simulink model "actuator_models"  (R2024b)
settings: Solver=FixedStepAuto  StartTime=0.0  StopTime=3  FixedStep=0.0001  RelTol=1e-3
libraries: aerolibactuator x4
settings Model: Creator=jonno  LastModifiedBy=jonno

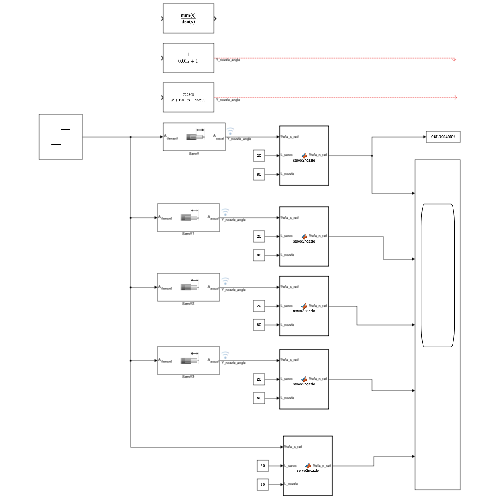
[thumbnail: Simulink's stored preview of the top-level diagram]
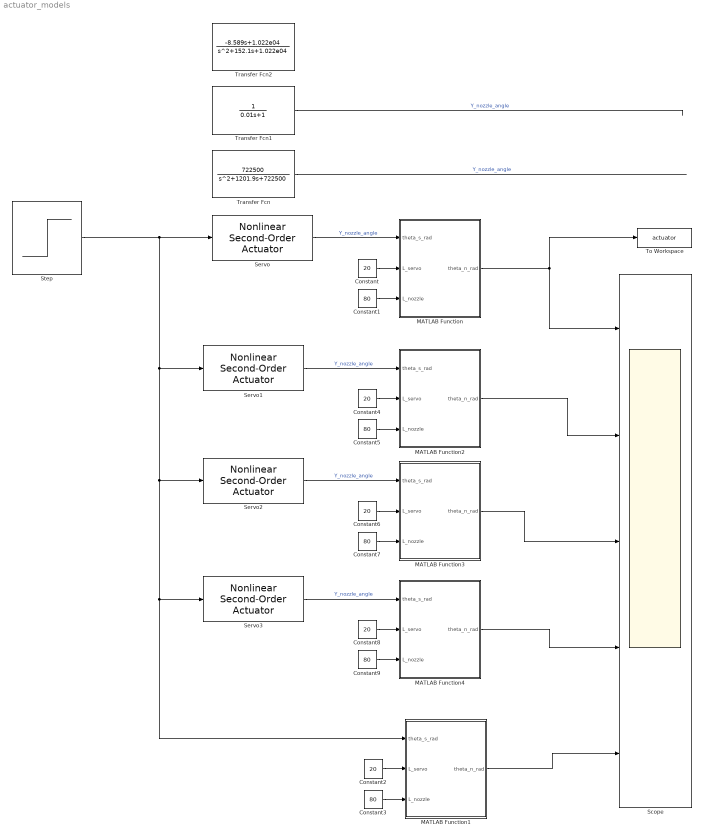
== system actuator_models ==
  Constant{,2,4,6,8} (5 alike) : Constant  Value=20
  Constant{1,3,5,7,9} (5 alike) : Constant  Value=80
  MATLAB Function : MATLAB Function  TreatAsAtomicUnit=on
  MATLAB Function1 : MATLAB Function  TreatAsAtomicUnit=on
  MATLAB Function2 : MATLAB Function  TreatAsAtomicUnit=on
  MATLAB Function3 : MATLAB Function  TreatAsAtomicUnit=on
  MATLAB Function4 : MATLAB Function  TreatAsAtomicUnit=on
  Scope : Scope  NumInputPorts=5
  Servo : aerolibactuator/Nonlinear Second-Order Actuator  wn_fin=60*10  z_fin=0.707  fin_max=60*pi/180  fin_min=-60*pi/180  fin_maxrate=(300*pi/180)*10  fin_act_0=0  fin_act_vel=0
  Servo1 : aerolibactuator/Nonlinear Second-Order Actuator  wn_fin=60*1  z_fin=0.707  fin_max=60*pi/180  fin_min=-60*pi/180  fin_maxrate=(300*pi/180)*10  fin_act_0=0  fin_act_vel=0
  Servo2 : aerolibactuator/Nonlinear Second-Order Actuator  wn_fin=60*10  z_fin=0.707  fin_max=60*pi/180  fin_min=-60*pi/180  fin_maxrate=(300*pi/180)*1  fin_act_0=0  fin_act_vel=0
  Servo3 : aerolibactuator/Nonlinear Second-Order Actuator  wn_fin=60*1  z_fin=0.707  fin_max=60*pi/180  fin_min=-60*pi/180  fin_maxrate=(300*pi/180)*1  fin_act_0=0  fin_act_vel=0
  Step : Step  Time=2  After=0.87266  SampleTime=0
  To Workspace : ToWorkspace  VariableName=actuator  SaveFormat=Timeseries  SampleTime=-1
  Transfer Fcn : TransferFcn  Numerator=[722500]  Denominator=[1 1201.9 722500]
  Transfer Fcn1 : TransferFcn  Denominator=[0.01 1]
  Transfer Fcn2 : TransferFcn  Numerator=[-8.589 1.022e04]  Denominator=[1 152.1 1.022e04]
  wires:
  Step/1 -> Servo1/1, Servo3/1, MATLAB Function1/1(theta_s_rad), Servo2/1, Servo/1
  Transfer Fcn/1 -> ?  "Y_nozzle_angle"
  Servo/1 -> MATLAB Function/1(theta_s_rad)  "Y_nozzle_angle"
  Transfer Fcn1/1 -> ?  "Y_nozzle_angle"
  MATLAB Function/1(theta_n_rad) -> To Workspace/1, Scope/1
  Constant/1 -> MATLAB Function/2(L_servo)
  Constant1/1 -> MATLAB Function/3(L_nozzle)
  Constant3/1 -> MATLAB Function1/3(L_nozzle)
  Constant2/1 -> MATLAB Function1/2(L_servo)
  MATLAB Function1/1(theta_n_rad) -> Scope/5
  Constant5/1 -> MATLAB Function2/3(L_nozzle)
  Servo1/1 -> MATLAB Function2/1(theta_s_rad)  "Y_nozzle_angle"
  MATLAB Function2/1(theta_n_rad) -> Scope/2
  Constant4/1 -> MATLAB Function2/2(L_servo)
  Constant6/1 -> MATLAB Function3/2(L_servo)
  Constant7/1 -> MATLAB Function3/3(L_nozzle)
  Servo2/1 -> MATLAB Function3/1(theta_s_rad)  "Y_nozzle_angle"
  Constant9/1 -> MATLAB Function4/3(L_nozzle)
  Constant8/1 -> MATLAB Function4/2(L_servo)
  Servo3/1 -> MATLAB Function4/1(theta_s_rad)  "Y_nozzle_angle"
  MATLAB Function3/1(theta_n_rad) -> Scope/3
  MATLAB Function4/1(theta_n_rad) -> Scope/4

== matlab function actuator_models/MATLAB Function ==
  data: theta_s_rad input; theta_n_rad output; L_servo input; L_nozzle input
function theta_n_rad = servo2nozzle(theta_s_rad, L_servo, L_nozzle)
    theta_n_rad = asin((L_servo / L_nozzle) * sin(theta_s_rad));
end

== matlab function actuator_models/MATLAB Function2 ==
  data: theta_s_rad input; theta_n_rad output; L_servo input; L_nozzle input
function theta_n_rad = servo2nozzle(theta_s_rad, L_servo, L_nozzle)
    theta_n_rad = asin((L_servo / L_nozzle) * sin(theta_s_rad));
end

== matlab function actuator_models/MATLAB Function3 ==
  data: theta_s_rad input; theta_n_rad output; L_servo input; L_nozzle input
function theta_n_rad = servo2nozzle(theta_s_rad, L_servo, L_nozzle)
    theta_n_rad = asin((L_servo / L_nozzle) * sin(theta_s_rad));
end

== matlab function actuator_models/MATLAB Function4 ==
  data: theta_s_rad input; theta_n_rad output; L_servo input; L_nozzle input
function theta_n_rad = servo2nozzle(theta_s_rad, L_servo, L_nozzle)
    theta_n_rad = asin((L_servo / L_nozzle) * sin(theta_s_rad));
end

== matlab function actuator_models/MATLAB Function1 ==
  data: theta_s_rad input; theta_n_rad output; L_servo input; L_nozzle input
function theta_n_rad = servo2nozzle(theta_s_rad, L_servo, L_nozzle)
    theta_n_rad = asin((L_servo / L_nozzle) * sin(theta_s_rad));
end
